simulink model "Solution_02"  (R2018b)
settings: Solver=VariableStepAuto  StartTime=0.0  StopTime=10.0  RelTol=1e-3
settings Model: Creator=Gowtham  LastModifiedBy=Gowtham

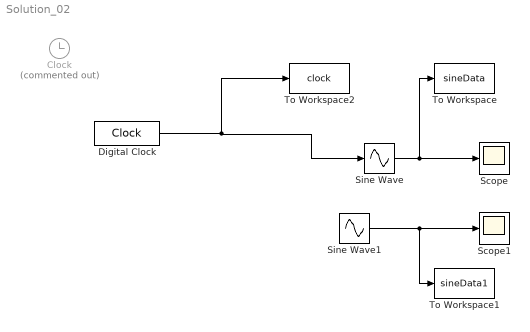
== system Solution_02 ==
  Clock : Clock  Commented=on
      settings: Decimation=100
  Digital Clock : DigitalClock  SampleTime=0.5
  Scope : Scope
  Scope1 : Scope
  Sine Wave : Sin  SineType=Sample based  TimeSource=Use external signal  SampleTime=0.01
  Sine Wave1 : Sin  SampleTime=0.01
  To Workspace : ToWorkspace  VariableName=sineData  SaveFormat=Timeseries  SampleTime=-1
  To Workspace1 : ToWorkspace  VariableName=sineData1  SaveFormat=Timeseries  SampleTime=-1
  To Workspace2 : ToWorkspace  VariableName=clock  SaveFormat=Timeseries  SampleTime=-1
  wires:
  Sine Wave/1 -> To Workspace/1, Scope/1
  Sine Wave1/1 -> To Workspace1/1, Scope1/1
  Digital Clock/1 -> Sine Wave/1, To Workspace2/1
